simulink model "flightController"  (R2022a)
settings: Solver=ode3  StartTime=0  StopTime=TFinal  FixedStep=Ts  RelTol=1e-3  EnableMultiTasking=on
undefined symbols (not defined in the file): Controller, DiscIntNeverNeededParam, Ts, Vehicle
libraries: vrlib x2, dspfdesign x1
(part 1 of 2)
settings Model: Creator=The MathWorks, Inc.  LastModifiedBy=martin
settings SolverCC: AlgebraicLoopSolver=TrustRegion  MinimalZcImpactIntegration=on
settings DataIOCC: LimitDataPoints=on  SaveFormat=Array  ReturnWorkspaceOutputs=off
settings OptimizationCC: BlockReduction=off  DefaultParameterBehavior=Inlined  BufferReuse=off  PassReuseOutputArgsThreshold=0
settings DebuggingCC: AlgebraicLoopMsg=none  ParameterPrecisionLossMsg=none  ParameterTunabilityLossMsg=error  BusObjectLabelMismatch=error  SFUnexpectedBacktrackingDiag=warning  SFNoUnconditionalDefaultTransitionDiag=warning  SFExecutionAtInitializationDiag=none  SFMachineParentedDataDiag=warning  ArithmeticOperatorsInVariantConditions=warning
settings HardwareCC: ProdBitPerPointer=32  ProdBitPerSizeT=32  ProdBitPerPtrDiffT=32  ProdLargestAtomicInteger=Long  ProdWordSize=32  ProdHWDeviceType=ARM Compatible->ARM 9
settings ModelReferenceCC: ModelReferenceNumInstancesAllowed=Single  PropagateSignalLabelsOutOfModel=off
settings SFSimCC: SimUseLocalCustomCode=off  CustomCodeUndefinedFunction=UseInterfaceOnly
settings RTWCC: Description=Generic Real-Time Target  GenerateReport=on  RTWUseLocalCustomCode=off  LaunchReport=on  DLArmComputeVersion=19.05
settings CodeAppCC: ForceParamTrailComments=on  MaxIdLength=63  OperatorAnnotations=on  StateflowObjectComments=on  MATLABSourceComments=on
settings GRTTargetCC: TargetLangStandard=C89/C90 (ANSI)
settings ConfigComp: CovMetricSettings=dw  CovSaveCumulativeToWorkspaceVar=on  CovSaveSingleToWorkspaceVar=on  CovExternalEMLEnable=off  CovSFcnEnable=off

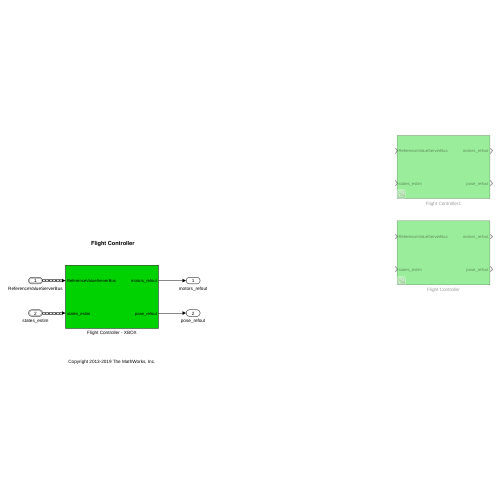
[thumbnail: Simulink's stored preview of the top-level diagram]
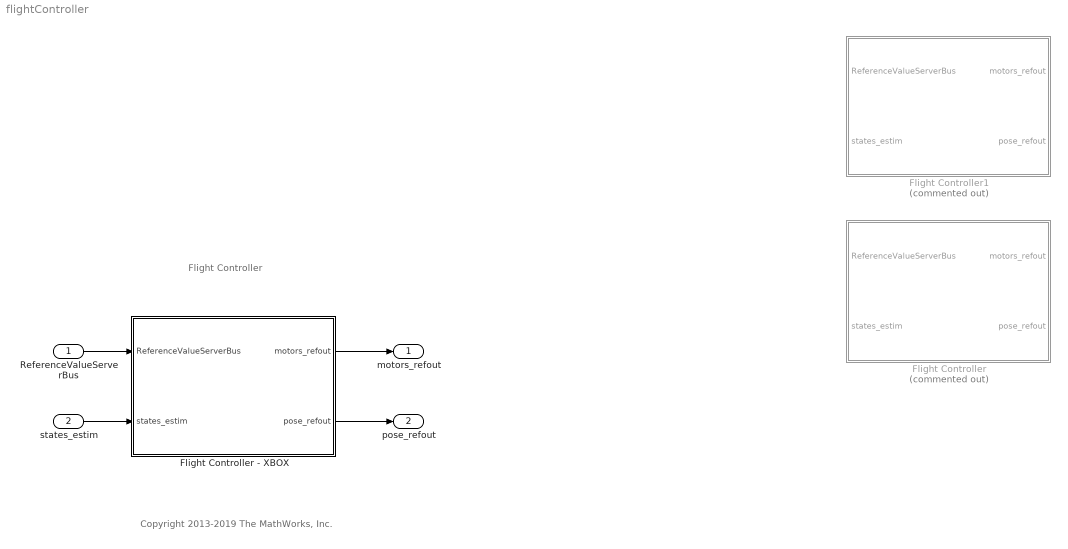
== system flightController ==
  note: Flight Controller
  note: Copyright 2013-2019 The MathWorks, Inc.
  ReferenceValueServerBus : Inport  OutDataTypeStr=Bus: CommandBus  BusOutputAsStruct=on
  states_estim : Inport  Port=2  OutDataTypeStr=Bus: statesEstim_t  BusOutputAsStruct=on
  Flight Controller : Subsystem  Commented=on
  Flight Controller - XBOX : Subsystem
  Flight Controller1 : Subsystem  Commented=on
  motors_refout : Outport  VectorParamsAs1DForOutWhenUnconnected=off
  pose_refout : Outport  Port=2  VectorParamsAs1DForOutWhenUnconnected=off
  wires:
  ReferenceValueServerBus/1 -> Flight Controller - XBOX/1(ReferenceValueServerBus)
  states_estim/1 -> Flight Controller - XBOX/2(states_estim)
  Flight Controller - XBOX/2(pose_refout) -> pose_refout/1
  Flight Controller - XBOX/1(motors_refout) -> motors_refout/1

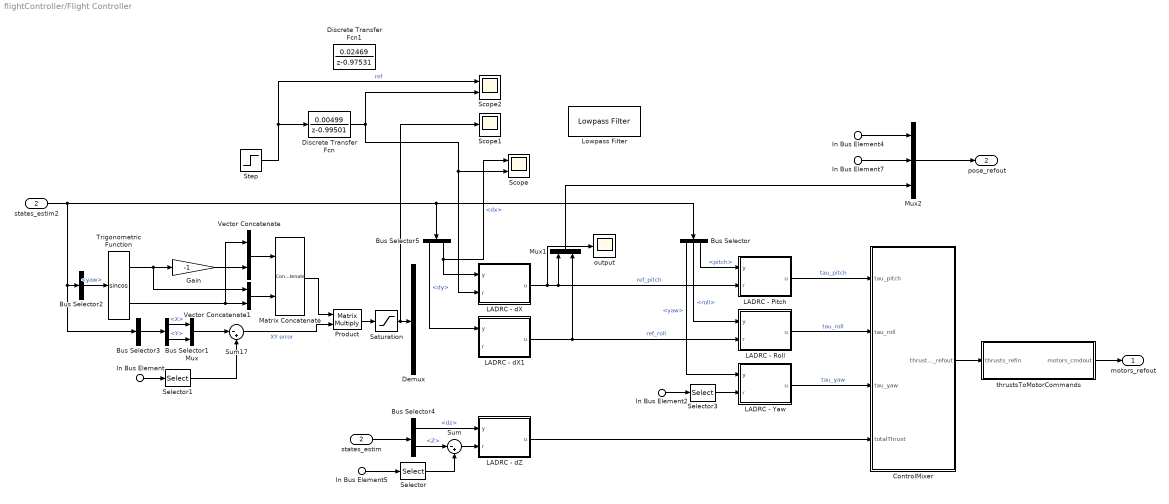
== system flightController/Flight Controller ==
  In Bus Element4 : Inport  PortName=ReferenceValueServerBus  Element=pos_ref
  In Bus Element5 : Inport  PortName=ReferenceValueServerBus  Element=pos_ref
  In Bus Element : Inport  PortName=ReferenceValueServerBus  Element=pos_ref
  In Bus Element2 : Inport  PortName=ReferenceValueServerBus  Element=orient_ref
  In Bus Element7 : Inport  PortName=ReferenceValueServerBus  Element=orient_ref
  states_estim : Inport  Port=2
  Bus Selector : BusSelector  OutputSignals=yaw,roll,pitch
  Bus Selector1 : BusSelector  OutputSignals=X,Y
  Bus Selector2 : BusSelector  OutputSignals=yaw
  Bus Selector3 : BusSelector  OutputSignals=X,Y  OutputAsBus=on
  Bus Selector4 : BusSelector  OutputSignals=dz,Z
  Bus Selector5 : BusSelector  OutputSignals=dy,dx
  ControlMixer : Subsystem
  Demux : Demux  Outputs=2
  Discrete Transfer Fcn : DiscreteTransferFcn  Numerator=[0.00499]  Denominator=[1 -0.99501]
  Discrete Transfer Fcn1 : DiscreteTransferFcn  Numerator=[0.02469]  Denominator=[1 -0.97531]
  Gain : Gain  Gain=-1
  LADRC - Pitch : Subsystem  VariantControl=Choice
  LADRC - Roll : Subsystem  VariantControl=Choice
  LADRC - Yaw : Subsystem  VariantControl=Choice
  LADRC - dX : Subsystem  VariantControl=Choice
  LADRC - dX1 : Subsystem  VariantControl=Choice
  LADRC - dZ : Subsystem  VariantControl=Choice
  Lowpass Filter : dspfdesign/Lowpass Filter  FilterType=IIR  DesignForMinimumOrder=off  FilterOrder=1  PassbandFrequency=4  StopbandFrequency=12e3  PassbandRipple=0.1  StopbandAttenuation=80  InheritSampleRate=off  SampleRate=200  SimulateUsing=Interpreted execution  roundingMode=Floor  coeffsDataTypeStr=fixdt(1,16)
  Matrix Concatenate : Concatenate  Mode=Multidimensional array  ConcatenateDimension=2
  Mux : Mux  Inputs=2
  Mux1 : Mux  Inputs=2
  Mux2 : Mux  Inputs=3
  Product : Product  Multiplication=Matrix(*)  OutDataTypeStr=single  RndMeth=Zero
  Saturation : Saturate  UpperLimit=3  LowerLimit=-3  OutDataTypeStr=single
  Scope : Scope  NumInputPorts=2
  Scope1 : Scope
  Scope2 : Scope  NumInputPorts=2
  Selector : Selector  InputPortWidth=3  IndexOptions=Index vector (dialog)  Indices=3  OutputSizes=1
  Selector1 : Selector  InputPortWidth=3  IndexOptions=Index vector (dialog)  Indices=[1 2]  OutputSizes=1
  Selector3 : Selector  InputPortWidth=3  IndexOptions=Index vector (dialog)  Indices=1  OutputSizes=1
  Step : Step  Time=5  After=0.5  SampleTime=Ts
  Sum : Sum  Inputs=|-+
  Sum17 : Sum  Inputs=|-+  AccumDataTypeStr=single
  Trigonometric Function : Trigonometry  Operator=sincos
  Vector Concatenate : Concatenate
  Vector Concatenate1 : Concatenate
  output : Scope
  states_estim2 : InportShadow  Port=2
  thrustsToMotorCommands : Subsystem
  motors_refout : Outport  VectorParamsAs1DForOutWhenUnconnected=off
  pose_refout : Outport  Port=2  VectorParamsAs1DForOutWhenUnconnected=off
  wires:
  thrustsToMotorCommands/1(motors_cmdout) -> motors_refout/1
  Mux2/1 -> pose_refout/1
  LADRC - dZ/1(u) -> ControlMixer/4(totalThrust)
  In Bus Element2/1 -> Selector3/1
  ControlMixer/1(thrusts_refout) -> thrustsToMotorCommands/1(thrusts_refin)
  Bus Selector5/2 -> Scope/1, LADRC - dX/1(y)  "<dx>"
  Bus Selector5/1 -> LADRC - dX1/1(y)  "<dy>"
  In Bus Element7/1 -> Mux2/2
  Selector3/1 -> LADRC - Yaw/2(r)
  Bus Selector4/1 -> LADRC - dZ/1(y)  "<dz>"
  In Bus Element5/1 -> Selector/1
  In Bus Element4/1 -> Mux2/1
  states_estim/1 -> Bus Selector4/1
  LADRC - Yaw/1(u) -> ControlMixer/3(tau_yaw)  "tau_yaw"
  Bus Selector/2 -> LADRC - Roll/1(y)  "<roll>"
  Bus Selector/3 -> LADRC - Pitch/1(y)  "<pitch>"
  LADRC - dX/1(u) -> output/1, LADRC - Pitch/2(r), Mux1/1  "ref_pitch"
  LADRC - Roll/1(u) -> ControlMixer/2(tau_roll)  "tau_roll"
  LADRC - dX1/1(u) -> LADRC - Roll/2(r), Mux1/2  "ref_roll"
  Mux1/1 -> Mux2/3
  LADRC - Pitch/1(u) -> ControlMixer/1(tau_pitch)  "tau_pitch"
  Bus Selector/1 -> LADRC - Yaw/1(y)  "<yaw>"
  Sum/1 -> LADRC - dZ/2(r)
  Bus Selector4/2 -> Sum/1  "<Z>"
  Selector/1 -> Sum/2
  Trigonometric Function/1 -> Gain/1, Vector Concatenate1/1
  Bus Selector3/1 -> Bus Selector1/1
  Bus Selector1/2 -> Mux/2  "<Y>"
  Mux/1 -> Sum17/1
  Sum17/1 -> Product/2  "XY error"
  Matrix Concatenate/1 -> Product/1
  Trigonometric Function/2 -> Vector Concatenate1/2, Vector Concatenate/1
  Bus Selector1/1 -> Mux/1  "<X>"
  Vector Concatenate1/1 -> Matrix Concatenate/2
  Bus Selector2/1 -> Trigonometric Function/1  "<yaw>"
  Gain/1 -> Vector Concatenate/2
  Product/1 -> Saturation/1
  Vector Concatenate/1 -> Matrix Concatenate/1
  states_estim2/1 -> Bus Selector/1, Bus Selector5/1, Bus Selector2/1, Bus Selector3/1
  In Bus Element/1 -> Selector1/1
  Selector1/1 -> Sum17/2
  Saturation/1 -> Scope1/1, Demux/1
  Step/1 -> Scope2/1, Discrete Transfer Fcn/1  "ref"
  ? -> LADRC - dX1/2(r)
  Discrete Transfer Fcn/1 -> Scope/2, LADRC - dX/2(r), Scope2/2

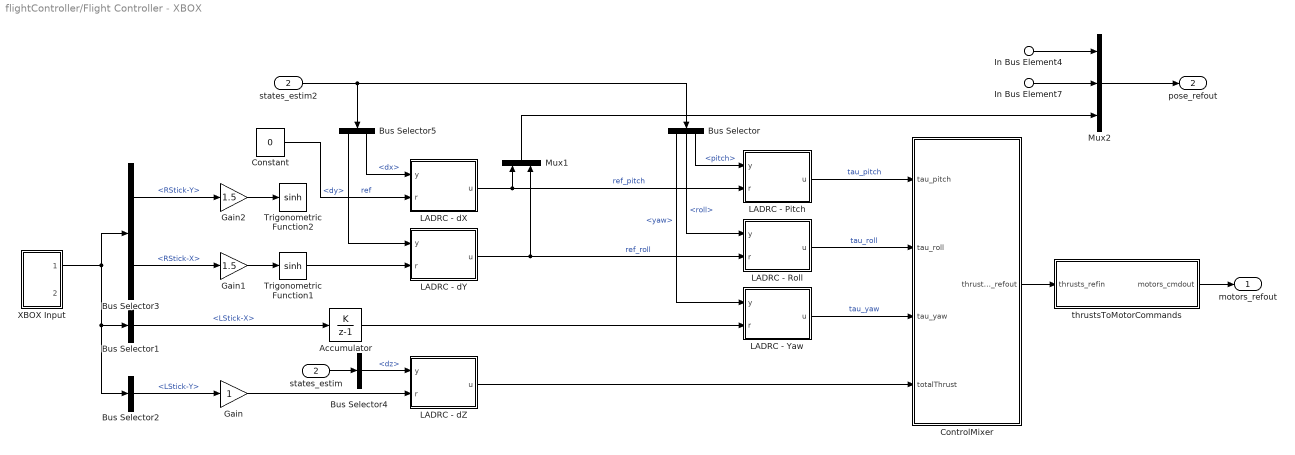
== system flightController/Flight Controller - XBOX ==
  In Bus Element4 : Inport  PortName=ReferenceValueServerBus  Element=pos_ref
  In Bus Element7 : Inport  PortName=ReferenceValueServerBus  Element=orient_ref
  states_estim : Inport  Port=2
  Accumulator : DiscreteIntegrator  IntegratorMethod=Accumulation: Forward Euler  gainval=0.01  SampleTime=-1  ICPrevOutput=DiscIntNeverNeededParam  ICPrevScaledInput=DiscIntNeverNeededParam
  Bus Selector : BusSelector  OutputSignals=yaw,roll,pitch
  Bus Selector1 : BusSelector  OutputSignals=LStick-X
  Bus Selector2 : BusSelector  OutputSignals=LStick-Y
  Bus Selector3 : BusSelector  OutputSignals=RStick-Y,RStick-X
  Bus Selector4 : BusSelector  OutputSignals=dz
  Bus Selector5 : BusSelector  OutputSignals=dy,dx
  Constant : Constant  Value=0  OutDataTypeStr=single  SampleTime=Ts
  ControlMixer : Subsystem
  Gain : Gain  OutDataTypeStr=single
  Gain1 : Gain  Gain=1.5  OutDataTypeStr=single
  Gain2 : Gain  Gain=1.5  OutDataTypeStr=single
  LADRC - Pitch : Subsystem  VariantControl=Choice
  LADRC - Roll : Subsystem  VariantControl=Choice
  LADRC - Yaw : Subsystem  VariantControl=Choice
  LADRC - dX : Subsystem  VariantControl=Choice
  LADRC - dY : Subsystem  VariantControl=Choice
  LADRC - dZ : Subsystem  VariantControl=Choice
  Mux1 : Mux  Inputs=2
  Mux2 : Mux  Inputs=3
  Trigonometric Function1 : Trigonometry  Operator=sinh
  Trigonometric Function2 : Trigonometry  Operator=sinh
  XBOX Input : Subsystem
  states_estim2 : InportShadow  Port=2
  thrustsToMotorCommands : Subsystem
  motors_refout : Outport  VectorParamsAs1DForOutWhenUnconnected=off
  pose_refout : Outport  Port=2  VectorParamsAs1DForOutWhenUnconnected=off
  wires:
  XBOX Input/1(Analog) -> Bus Selector3/1, Bus Selector2/1, Bus Selector1/1
  thrustsToMotorCommands/1(motors_cmdout) -> motors_refout/1
  Mux2/1 -> pose_refout/1
  ControlMixer/1(thrusts_refout) -> thrustsToMotorCommands/1(thrusts_refin)
  Constant/1 -> LADRC - dX/2(r)  "ref"
  Bus Selector3/2 -> Gain1/1  "<RStick-X>"
  Bus Selector5/2 -> LADRC - dX/1(y)  "<dx>"
  Gain2/1 -> Trigonometric Function2/1
  Bus Selector3/1 -> Gain2/1  "<RStick-Y>"
  Bus Selector5/1 -> LADRC - dY/1(y)  "<dy>"
  Accumulator/1 -> LADRC - Yaw/2(r)
  In Bus Element7/1 -> Mux2/2
  Bus Selector4/1 -> LADRC - dZ/1(y)  "<dz>"
  Bus Selector2/1 -> Gain/1  "<LStick-Y>"
  Gain1/1 -> Trigonometric Function1/1
  In Bus Element4/1 -> Mux2/1
  Bus Selector1/1 -> Accumulator/1  "<LStick-X>"
  LADRC - Yaw/1(u) -> ControlMixer/3(tau_yaw)  "tau_yaw"
  Bus Selector/2 -> LADRC - Roll/1(y)  "<roll>"
  Bus Selector/3 -> LADRC - Pitch/1(y)  "<pitch>"
  LADRC - dX/1(u) -> LADRC - Pitch/2(r), Mux1/1  "ref_pitch"
  LADRC - Roll/1(u) -> ControlMixer/2(tau_roll)  "tau_roll"
  LADRC - dY/1(u) -> LADRC - Roll/2(r), Mux1/2  "ref_roll"
  Mux1/1 -> Mux2/3
  states_estim2/1 -> Bus Selector/1, Bus Selector5/1
  LADRC - Pitch/1(u) -> ControlMixer/1(tau_pitch)  "tau_pitch"
  Bus Selector/1 -> LADRC - Yaw/1(y)  "<yaw>"
  states_estim/1 -> Bus Selector4/1
  LADRC - dZ/1(u) -> ControlMixer/4(totalThrust)
  Trigonometric Function1/1 -> LADRC - dY/2(r)
  Gain/1 -> LADRC - dZ/2(r)

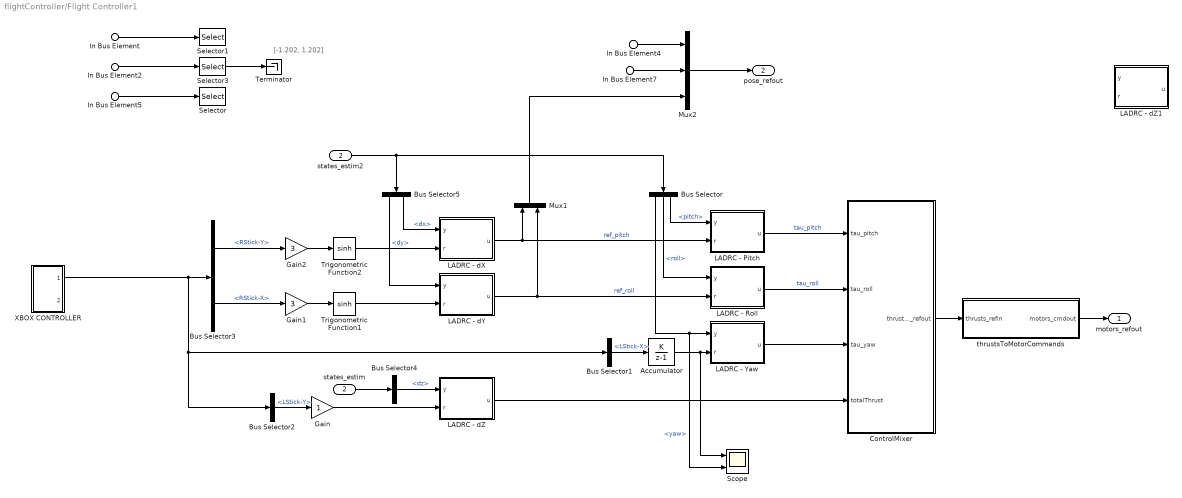
== system flightController/Flight Controller1 ==
  note: [-1.202, 1.202]
  In Bus Element : Inport  PortName=ReferenceValueServerBus  Element=pos_ref
  In Bus Element4 : Inport  PortName=ReferenceValueServerBus  Element=pos_ref
  In Bus Element5 : Inport  PortName=ReferenceValueServerBus  Element=pos_ref
  In Bus Element2 : Inport  PortName=ReferenceValueServerBus  Element=orient_ref
  In Bus Element7 : Inport  PortName=ReferenceValueServerBus  Element=orient_ref
  states_estim : Inport  Port=2
  Accumulator : DiscreteIntegrator  IntegratorMethod=Accumulation: Forward Euler  gainval=0.01  SampleTime=-1  ICPrevOutput=DiscIntNeverNeededParam  ICPrevScaledInput=DiscIntNeverNeededParam
  Bus Selector : BusSelector  OutputSignals=yaw,roll,pitch
  Bus Selector1 : BusSelector  OutputSignals=LStick-X
  Bus Selector2 : BusSelector  OutputSignals=LStick-Y
  Bus Selector3 : BusSelector  OutputSignals=RStick-Y,RStick-X
  Bus Selector4 : BusSelector  OutputSignals=dz
  Bus Selector5 : BusSelector  OutputSignals=dy,dx
  ControlMixer : Subsystem
  Gain : Gain  OutDataTypeStr=single
  Gain1 : Gain  Gain=3  OutDataTypeStr=single
  Gain2 : Gain  Gain=3  OutDataTypeStr=single
  LADRC - Pitch : Subsystem  VariantControl=Choice
  LADRC - Roll : Subsystem  VariantControl=Choice
  LADRC - Yaw : Subsystem  VariantControl=Choice
  LADRC - dX : Subsystem  VariantControl=Choice
  LADRC - dY : Subsystem  VariantControl=Choice
  LADRC - dZ : Subsystem  VariantControl=Choice
  LADRC - dZ1 : Subsystem  VariantControl=Choice
  Mux1 : Mux  Inputs=2
  Mux2 : Mux  Inputs=3
  Scope : Scope  NumInputPorts=2
  Selector : Selector  InputPortWidth=3  IndexOptions=Index vector (dialog)  Indices=3  OutputSizes=1
  Selector1 : Selector  InputPortWidth=3  IndexOptions=Index vector (dialog)  Indices=[1 2]  OutputSizes=1
  Selector3 : Selector  InputPortWidth=3  IndexOptions=Index vector (dialog)  Indices=1  OutputSizes=1
  Terminator : Terminator
  Trigonometric Function1 : Trigonometry  Operator=sinh
  Trigonometric Function2 : Trigonometry  Operator=sinh
  XBOX CONTROLLER : Subsystem
  states_estim2 : InportShadow  Port=2
  thrustsToMotorCommands : Subsystem
  motors_refout : Outport  VectorParamsAs1DForOutWhenUnconnected=off
  pose_refout : Outport  Port=2  VectorParamsAs1DForOutWhenUnconnected=off
  wires:
  XBOX CONTROLLER/1(Analog) -> Bus Selector2/1, Bus Selector1/1, Bus Selector3/1
  thrustsToMotorCommands/1(motors_cmdout) -> motors_refout/1
  Mux2/1 -> pose_refout/1
  In Bus Element/1 -> Selector1/1
  LADRC - dZ/1(u) -> ControlMixer/4(totalThrust)
  In Bus Element2/1 -> Selector3/1
  ControlMixer/1(thrusts_refout) -> thrustsToMotorCommands/1(thrusts_refin)
  Trigonometric Function2/1 -> LADRC - dX/2(r)
  Bus Selector3/2 -> Gain1/1  "<RStick-X>"
  Bus Selector5/2 -> LADRC - dX/1(y)  "<dx>"
  Gain2/1 -> Trigonometric Function2/1
  Bus Selector3/1 -> Gain2/1  "<RStick-Y>"
  Trigonometric Function1/1 -> LADRC - dY/2(r)
  Bus Selector5/1 -> LADRC - dY/1(y)  "<dy>"
  Accumulator/1 -> LADRC - Yaw/2(r), Scope/1
  In Bus Element7/1 -> Mux2/2
  Selector3/1 -> Terminator/1
  Bus Selector4/1 -> LADRC - dZ/1(y)  "<dz>"
  Bus Selector2/1 -> Gain/1  "<LStick-Y>"
  In Bus Element5/1 -> Selector/1
  Gain1/1 -> Trigonometric Function1/1
  In Bus Element4/1 -> Mux2/1
  states_estim/1 -> Bus Selector4/1
  Bus Selector1/1 -> Accumulator/1  "<LStick-X>"
  LADRC - Yaw/1(u) -> ControlMixer/3(tau_yaw)
  Bus Selector/2 -> LADRC - Roll/1(y)  "<roll>"
  Bus Selector/3 -> LADRC - Pitch/1(y)  "<pitch>"
  LADRC - dX/1(u) -> LADRC - Pitch/2(r), Mux1/1  "ref_pitch"
  LADRC - Roll/1(u) -> ControlMixer/2(tau_roll)  "tau_roll"
  LADRC - dY/1(u) -> Mux1/2, LADRC - Roll/2(r)  "ref_roll"
  Mux1/1 -> Mux2/3
  states_estim2/1 -> Bus Selector/1, Bus Selector5/1
  LADRC - Pitch/1(u) -> ControlMixer/1(tau_pitch)  "tau_pitch"
  Bus Selector/1 -> LADRC - Yaw/1(y), Scope/2  "<yaw>"
  Gain/1 -> LADRC - dZ/2(r)

== system flightController/Flight Controller/ControlMixer ==
  tau_pitch : Inport
  tau_roll : Inport  Port=2
  tau_yaw : Inport  Port=3
  totalThrust : Inport  Port=4
  Mux2 : Mux
  Product : Product  Multiplication=Matrix(*)  RndMeth=Zero
  TorqueTotalThrustToThrustPerMotor : Constant  Value=Controller.Q2Ts  OutDataTypeStr=single
  thrusts_refout : Outport  VectorParamsAs1DForOutWhenUnconnected=off
  wires:
  Product/1 -> thrusts_refout/1
  tau_roll/1 -> Mux2/4
  tau_pitch/1 -> Mux2/3
  tau_yaw/1 -> Mux2/2
  totalThrust/1 -> Mux2/1
  TorqueTotalThrustToThrustPerMotor/1 -> Product/1
  Mux2/1 -> Product/2

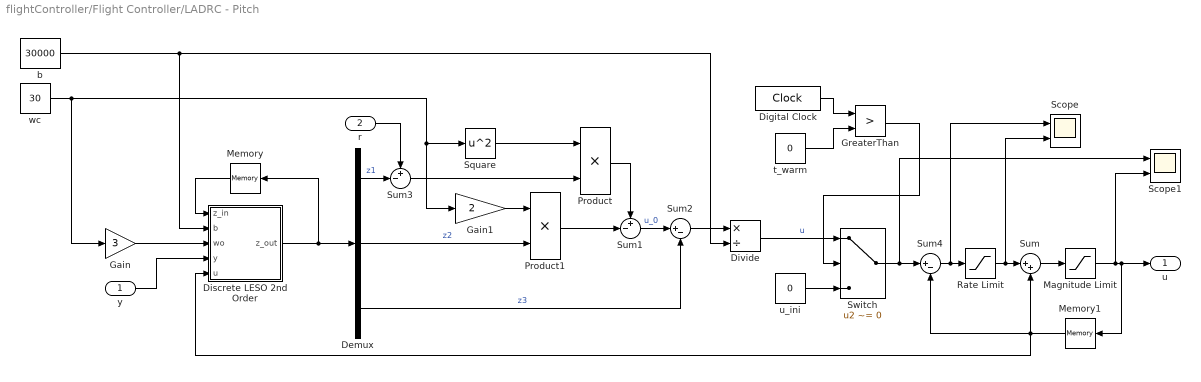
== system flightController/Flight Controller/LADRC - Pitch ==
  y : Inport
  r : Inport  Port=2
  Demux : Demux  Outputs=3
  Digital Clock : DigitalClock  SampleTime=Ts
  Discrete LESO 2nd Order : MATLAB Function  TreatAsAtomicUnit=on
  Divide : Product  Inputs=*/  OutDataTypeStr=single
  Gain : Gain  Gain=3  OutDataTypeStr=single
  Gain1 : Gain  Gain=2  OutDataTypeStr=single
  GreaterThan : RelationalOperator  Operator=>  OutDataTypeStr=boolean  RndMeth=Simplest  InputSameDT=off
  Magnitude Limit : Saturate  UpperLimit=4*Controller.totalThrustMaxRelative*Controller.motorsThrustPerMotorMax  LowerLimit=-4*Controller.totalThrustMaxRelative*Controller.motorsThrustPerMotorMax  OutDataTypeStr=single
  Memory : Memory  InitialCondition=[0 0 0]'
  Memory1 : Memory
  Product : Product  OutDataTypeStr=single
  Product1 : Product  OutDataTypeStr=single
  Rate Limit : Saturate  UpperLimit=0.05  LowerLimit=-0.05
  Scope : Scope  NumInputPorts=2
  Scope1 : Scope  NumInputPorts=2
  Square : Math  Operator=square
  Sum : Sum  Inputs=|++
  Sum1 : Sum  Inputs=+-|
  Sum2 : Sum  Inputs=|+-
  Sum3 : Sum  Inputs=+-|
  Sum4 : Sum  Inputs=|+-
  Switch : Switch  Criteria=u2 ~= 0  Threshold=0.1  SaturateOnIntegerOverflow=off  InputSameDT=off
  b : Constant  Value=30000  OutDataTypeStr=single
  t_warm : Constant  Value=0  OutDataTypeStr=single
  u_ini : Constant  Value=0  OutDataTypeStr=single
  wc : Constant  Value=30  OutDataTypeStr=single
  u : Outport
  wires:
  Discrete LESO 2nd Order/1(z_out) -> Memory/1, Demux/1
  Demux/1 -> Sum3/2  "z1"
  Product/1 -> Sum1/1
  Sum1/1 -> Sum2/1  "u_0"
  Demux/3 -> Sum2/2  "z3"
  Sum2/1 -> Divide/1
  Square/1 -> Product/1
  Gain1/1 -> Product1/1
  Demux/2 -> Product1/2  "z2"
  Product1/1 -> Sum1/2
  Divide/1 -> Switch/1  "u"
  u_ini/1 -> Switch/3
  r/1 -> Sum3/1
  Sum3/1 -> Product/2
  b/1 -> Divide/2, Discrete LESO 2nd Order/2(b)
  wc/1 -> Gain/1, Square/1, Gain1/1
  Gain/1 -> Discrete LESO 2nd Order/3(wo)
  t_warm/1 -> GreaterThan/2
  Digital Clock/1 -> GreaterThan/1
  GreaterThan/1 -> Switch/2
  y/1 -> Discrete LESO 2nd Order/4(y)
  Memory/1 -> Discrete LESO 2nd Order/1(z_in)
  Memory1/1 -> Sum4/2, Discrete LESO 2nd Order/5(u), Sum/2
  Rate Limit/1 -> Scope/2, Sum/1
  Sum/1 -> Magnitude Limit/1
  Sum4/1 -> Scope/1, Rate Limit/1
  Switch/1 -> Scope1/1, Sum4/1
  Magnitude Limit/1 -> Scope1/2, u/1, Memory1/1

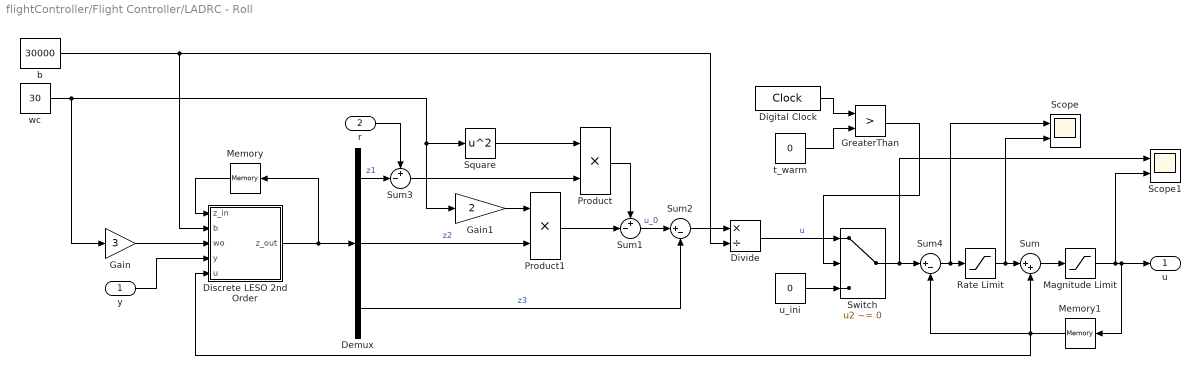
== system flightController/Flight Controller/LADRC - Roll ==
  y : Inport
  r : Inport  Port=2
  Demux : Demux  Outputs=3
  Digital Clock : DigitalClock  SampleTime=Ts
  Discrete LESO 2nd Order : MATLAB Function  TreatAsAtomicUnit=on
  Divide : Product  Inputs=*/  OutDataTypeStr=single
  Gain : Gain  Gain=3  OutDataTypeStr=single
  Gain1 : Gain  Gain=2  OutDataTypeStr=single
  GreaterThan : RelationalOperator  Operator=>  OutDataTypeStr=boolean  RndMeth=Simplest  InputSameDT=off
  Magnitude Limit : Saturate  UpperLimit=4*Controller.totalThrustMaxRelative*Controller.motorsThrustPerMotorMax  LowerLimit=-4*Controller.totalThrustMaxRelative*Controller.motorsThrustPerMotorMax  OutDataTypeStr=single
  Memory : Memory  InitialCondition=[0 0 0]'
  Memory1 : Memory
  Product : Product  OutDataTypeStr=single
  Product1 : Product  OutDataTypeStr=single
  Rate Limit : Saturate  UpperLimit=0.05  LowerLimit=-0.05
  Scope : Scope  NumInputPorts=2
  Scope1 : Scope  NumInputPorts=2
  Square : Math  Operator=square
  Sum : Sum  Inputs=|++
  Sum1 : Sum  Inputs=+-|
  Sum2 : Sum  Inputs=|+-
  Sum3 : Sum  Inputs=+-|
  Sum4 : Sum  Inputs=|+-
  Switch : Switch  Criteria=u2 ~= 0  Threshold=0.1  SaturateOnIntegerOverflow=off  InputSameDT=off
  b : Constant  Value=30000  OutDataTypeStr=single
  t_warm : Constant  Value=0  OutDataTypeStr=single
  u_ini : Constant  Value=0  OutDataTypeStr=single
  wc : Constant  Value=30  OutDataTypeStr=single
  u : Outport
  wires:
  Discrete LESO 2nd Order/1(z_out) -> Memory/1, Demux/1
  Demux/1 -> Sum3/2  "z1"
  Product/1 -> Sum1/1
  Sum1/1 -> Sum2/1  "u_0"
  Demux/3 -> Sum2/2  "z3"
  Sum2/1 -> Divide/1
  Square/1 -> Product/1
  Gain1/1 -> Product1/1
  Demux/2 -> Product1/2  "z2"
  Product1/1 -> Sum1/2
  Divide/1 -> Switch/1  "u"
  u_ini/1 -> Switch/3
  r/1 -> Sum3/1
  Sum3/1 -> Product/2
  b/1 -> Divide/2, Discrete LESO 2nd Order/2(b)
  wc/1 -> Gain/1, Square/1, Gain1/1
  Gain/1 -> Discrete LESO 2nd Order/3(wo)
  t_warm/1 -> GreaterThan/2
  Digital Clock/1 -> GreaterThan/1
  GreaterThan/1 -> Switch/2
  y/1 -> Discrete LESO 2nd Order/4(y)
  Memory/1 -> Discrete LESO 2nd Order/1(z_in)
  Memory1/1 -> Sum4/2, Discrete LESO 2nd Order/5(u), Sum/2
  Rate Limit/1 -> Scope/2, Sum/1
  Sum/1 -> Magnitude Limit/1
  Sum4/1 -> Scope/1, Rate Limit/1
  Switch/1 -> Scope1/1, Sum4/1
  Magnitude Limit/1 -> Scope1/2, u/1, Memory1/1

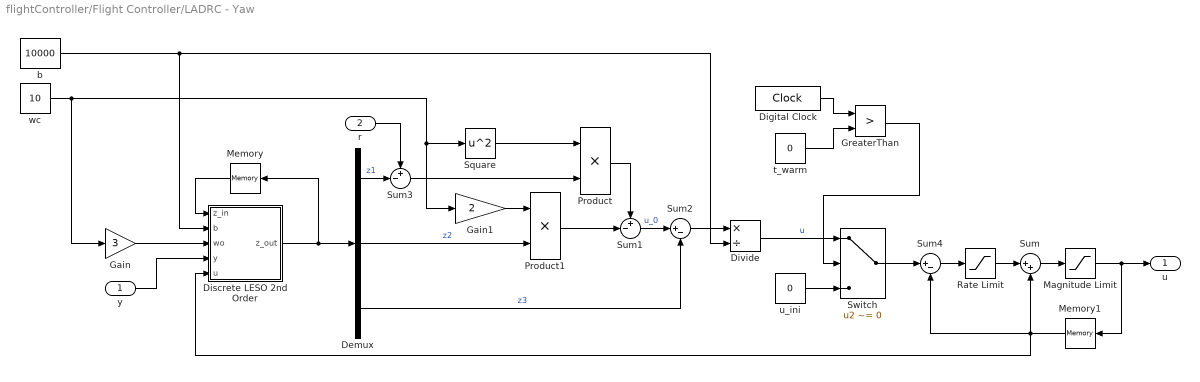
== system flightController/Flight Controller/LADRC - Yaw ==
  y : Inport
  r : Inport  Port=2
  Demux : Demux  Outputs=3
  Digital Clock : DigitalClock  SampleTime=Ts
  Discrete LESO 2nd Order : MATLAB Function  TreatAsAtomicUnit=on
  Divide : Product  Inputs=*/  OutDataTypeStr=single
  Gain : Gain  Gain=3  OutDataTypeStr=single
  Gain1 : Gain  Gain=2  OutDataTypeStr=single
  GreaterThan : RelationalOperator  Operator=>  OutDataTypeStr=boolean  RndMeth=Simplest  InputSameDT=off
  Magnitude Limit : Saturate  UpperLimit=4*Controller.totalThrustMaxRelative*Controller.motorsThrustPerMotorMax  LowerLimit=-4*Controller.totalThrustMaxRelative*Controller.motorsThrustPerMotorMax  OutDataTypeStr=single
  Memory : Memory  InitialCondition=[0 0 0]'
  Memory1 : Memory
  Product : Product  OutDataTypeStr=single
  Product1 : Product  OutDataTypeStr=single
  Rate Limit : Saturate  UpperLimit=0.05  LowerLimit=-0.05
  Square : Math  Operator=square
  Sum : Sum  Inputs=|++
  Sum1 : Sum  Inputs=+-|
  Sum2 : Sum  Inputs=|+-
  Sum3 : Sum  Inputs=+-|
  Sum4 : Sum  Inputs=|+-
  Switch : Switch  Criteria=u2 ~= 0  Threshold=0.1  SaturateOnIntegerOverflow=off  InputSameDT=off
  b : Constant  Value=10000  OutDataTypeStr=single
  t_warm : Constant  Value=0  OutDataTypeStr=single
  u_ini : Constant  Value=0  OutDataTypeStr=single
  wc : Constant  Value=10  OutDataTypeStr=single
  u : Outport
  wires:
  Discrete LESO 2nd Order/1(z_out) -> Memory/1, Demux/1
  Demux/1 -> Sum3/2  "z1"
  Product/1 -> Sum1/1
  Sum1/1 -> Sum2/1  "u_0"
  Demux/3 -> Sum2/2  "z3"
  Sum2/1 -> Divide/1
  Square/1 -> Product/1
  Gain1/1 -> Product1/1
  Demux/2 -> Product1/2  "z2"
  Product1/1 -> Sum1/2
  Divide/1 -> Switch/1  "u"
  u_ini/1 -> Switch/3
  r/1 -> Sum3/1
  Sum3/1 -> Product/2
  b/1 -> Divide/2, Discrete LESO 2nd Order/2(b)
  wc/1 -> Gain/1, Square/1, Gain1/1
  Gain/1 -> Discrete LESO 2nd Order/3(wo)
  t_warm/1 -> GreaterThan/2
  Digital Clock/1 -> GreaterThan/1
  GreaterThan/1 -> Switch/2
  y/1 -> Discrete LESO 2nd Order/4(y)
  Memory/1 -> Discrete LESO 2nd Order/1(z_in)
  Memory1/1 -> Sum4/2, Discrete LESO 2nd Order/5(u), Sum/2
  Rate Limit/1 -> Sum/1
  Sum/1 -> Magnitude Limit/1
  Sum4/1 -> Rate Limit/1
  Switch/1 -> Sum4/1
  Magnitude Limit/1 -> u/1, Memory1/1

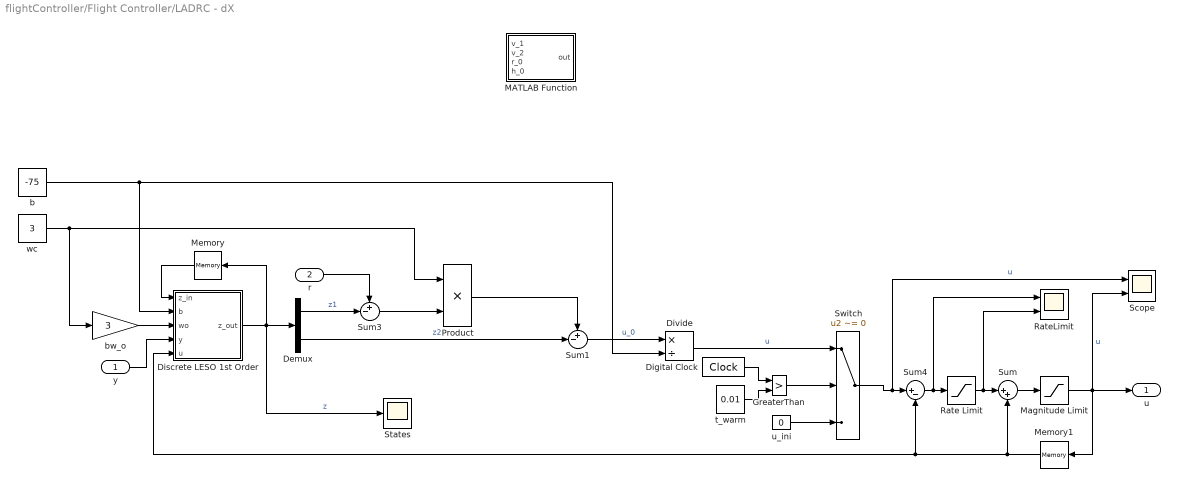
== system flightController/Flight Controller/LADRC - dX ==
  y : Inport
  r : Inport  Port=2
  Demux : Demux  Outputs=2
  Digital Clock : DigitalClock  SampleTime=Ts
  Discrete LESO 1st Order : MATLAB Function  TreatAsAtomicUnit=on
  Divide : Product  Inputs=*/
  GreaterThan : RelationalOperator  Operator=>  OutDataTypeStr=boolean  RndMeth=Simplest  InputSameDT=off
  MATLAB Function : MATLAB Function  TreatAsAtomicUnit=on
  Magnitude Limit : Saturate  UpperLimit=pi/8  LowerLimit=-pi/8  OutDataTypeStr=single
  Memory : Memory  InitialCondition=[0 0]'
  Memory1 : Memory
  Product : Product
  Rate Limit : Saturate  UpperLimit=0.2  LowerLimit=-0.2
  RateLimit : Scope  NumInputPorts=2
  Scope : Scope  NumInputPorts=2
  States : Scope
  Sum : Sum  Inputs=|++
  Sum1 : Sum  Inputs=+-|
  Sum3 : Sum  Inputs=+-|
  Sum4 : Sum  Inputs=|+-
  Switch : Switch  Criteria=u2 ~= 0  Threshold=0.1  SaturateOnIntegerOverflow=off  InputSameDT=off
  b : Constant  Value=-75  OutDataTypeStr=single
  bw_o : Gain  Gain=3
  t_warm : Constant  Value=0.01
  u_ini : Constant  Value=0  OutDataTypeStr=single
  wc : Constant  Value=3  OutDataTypeStr=single
  u : Outport
  wires:
  Demux/1 -> Sum3/2  "z1"
  Product/1 -> Sum1/1
  Sum1/1 -> Divide/1  "u_0"
  Demux/2 -> Sum1/2  "z2"
  Magnitude Limit/1 -> Scope/2, u/1, Memory1/1  "u"
  Divide/1 -> Switch/1  "u"
  u_ini/1 -> Switch/3
  r/1 -> Sum3/1
  Sum3/1 -> Product/2
  b/1 -> Divide/2, Discrete LESO 1st Order/2(b)
  wc/1 -> Product/1, bw_o/1
  bw_o/1 -> Discrete LESO 1st Order/3(wo)
  t_warm/1 -> GreaterThan/2
  Digital Clock/1 -> GreaterThan/1
  GreaterThan/1 -> Switch/2
  y/1 -> Discrete LESO 1st Order/4(y)
  Switch/1 -> Scope/1, Sum4/1  "u"
  Discrete LESO 1st Order/1(z_out) -> States/1, Memory/1, Demux/1  "z"
  Memory/1 -> Discrete LESO 1st Order/1(z_in)
  Rate Limit/1 -> RateLimit/2, Sum/1
  Memory1/1 -> Discrete LESO 1st Order/5(u), Sum4/2, Sum/2
  Sum4/1 -> RateLimit/1, Rate Limit/1
  Sum/1 -> Magnitude Limit/1

== system flightController/Flight Controller/LADRC - dX1 ==
  y : Inport
  r : Inport  Port=2
  Demux : Demux  Outputs=2
  Digital Clock : DigitalClock  SampleTime=Ts
  Discrete LESO 1st Order : MATLAB Function  TreatAsAtomicUnit=on
  Divide : Product  Inputs=*/
  GreaterThan : RelationalOperator  Operator=>  OutDataTypeStr=boolean  RndMeth=Simplest  InputSameDT=off
  Magnitude Limit : Saturate  UpperLimit=pi/8  LowerLimit=-pi/8  OutDataTypeStr=single
  Memory : Memory  InitialCondition=[0 0]'
  Memory1 : Memory
  Product : Product
  Rate Limit : Saturate  UpperLimit=1  LowerLimit=-1
  Sum : Sum  Inputs=|++
  Sum1 : Sum  Inputs=+-|
  Sum3 : Sum  Inputs=+-|
  Sum4 : Sum  Inputs=|+-
  Switch : Switch  Criteria=u2 ~= 0  Threshold=0.1  SaturateOnIntegerOverflow=off  InputSameDT=off
  b : Constant  Value=60  OutDataTypeStr=single
  bw_o : Gain  Gain=3
  t_warm : Constant  Value=0.01
  u_ini : Constant  Value=0  OutDataTypeStr=single
  wc : Constant  OutDataTypeStr=single
  u : Outport
  wires:
  Demux/1 -> Sum3/2  "z1"
  Product/1 -> Sum1/1
  Sum1/1 -> Divide/1  "u_0"
  Demux/2 -> Sum1/2  "z2"
  Magnitude Limit/1 -> u/1, Memory1/1  "u"
  Divide/1 -> Switch/1  "u"
  u_ini/1 -> Switch/3
  r/1 -> Sum3/1
  Sum3/1 -> Product/2
  b/1 -> Divide/2, Discrete LESO 1st Order/2(b)
  wc/1 -> Product/1, bw_o/1
  bw_o/1 -> Discrete LESO 1st Order/3(wo)
  t_warm/1 -> GreaterThan/2
  Digital Clock/1 -> GreaterThan/1
  GreaterThan/1 -> Switch/2
  y/1 -> Discrete LESO 1st Order/4(y)
  Switch/1 -> Sum4/1  "u"
  Discrete LESO 1st Order/1(z_out) -> Memory/1, Demux/1
  Memory/1 -> Discrete LESO 1st Order/1(z_in)
  Rate Limit/1 -> Sum/1
  Memory1/1 -> Discrete LESO 1st Order/5(u), Sum4/2, Sum/2
  Sum4/1 -> Rate Limit/1
  Sum/1 -> Magnitude Limit/1

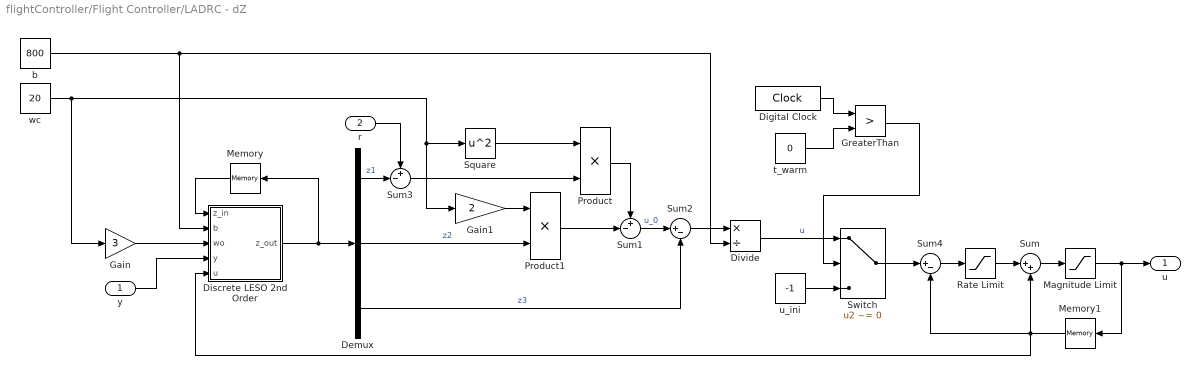
== system flightController/Flight Controller/LADRC - dZ ==
  y : Inport
  r : Inport  Port=2
  Demux : Demux  Outputs=3
  Digital Clock : DigitalClock  SampleTime=Ts
  Discrete LESO 2nd Order : MATLAB Function  TreatAsAtomicUnit=on
  Divide : Product  Inputs=*/  OutDataTypeStr=single
  Gain : Gain  Gain=3  OutDataTypeStr=single
  Gain1 : Gain  Gain=2  OutDataTypeStr=single
  GreaterThan : RelationalOperator  Operator=>  OutDataTypeStr=boolean  RndMeth=Simplest  InputSameDT=off
  Magnitude Limit : Saturate  UpperLimit=4*Controller.totalThrustMaxRelative*Controller.motorsThrustPerMotorMax  LowerLimit=-4*Controller.totalThrustMaxRelative*Controller.motorsThrustPerMotorMax  OutDataTypeStr=single
  Memory : Memory  InitialCondition=[0 0 380]'
  Memory1 : Memory  InitialCondition=-0.6
  Product : Product  OutDataTypeStr=single
  Product1 : Product  OutDataTypeStr=single
  Rate Limit : Saturate  UpperLimit=0.025  LowerLimit=-0.025
  Square : Math  Operator=square
  Sum : Sum  Inputs=|++
  Sum1 : Sum  Inputs=+-|
  Sum2 : Sum  Inputs=|+-
  Sum3 : Sum  Inputs=+-|
  Sum4 : Sum  Inputs=|+-
  Switch : Switch  Criteria=u2 ~= 0  Threshold=0.1  SaturateOnIntegerOverflow=off  InputSameDT=off
  b : Constant  Value=800  OutDataTypeStr=single
  t_warm : Constant  Value=0  OutDataTypeStr=single
  u_ini : Constant  Value=-1  OutDataTypeStr=single
  wc : Constant  Value=20  OutDataTypeStr=single
  u : Outport
  wires:
  Discrete LESO 2nd Order/1(z_out) -> Memory/1, Demux/1
  Demux/1 -> Sum3/2  "z1"
  Product/1 -> Sum1/1
  Sum1/1 -> Sum2/1  "u_0"
  Demux/3 -> Sum2/2  "z3"
  Sum2/1 -> Divide/1
  Square/1 -> Product/1
  Gain1/1 -> Product1/1
  Demux/2 -> Product1/2  "z2"
  Product1/1 -> Sum1/2
  Divide/1 -> Switch/1  "u"
  u_ini/1 -> Switch/3
  r/1 -> Sum3/1
  Sum3/1 -> Product/2
  b/1 -> Divide/2, Discrete LESO 2nd Order/2(b)
  wc/1 -> Gain/1, Square/1, Gain1/1
  Gain/1 -> Discrete LESO 2nd Order/3(wo)
  t_warm/1 -> GreaterThan/2
  Digital Clock/1 -> GreaterThan/1
  GreaterThan/1 -> Switch/2
  y/1 -> Discrete LESO 2nd Order/4(y)
  Memory/1 -> Discrete LESO 2nd Order/1(z_in)
  Memory1/1 -> Sum4/2, Discrete LESO 2nd Order/5(u), Sum/2
  Rate Limit/1 -> Sum/1
  Sum/1 -> Magnitude Limit/1
  Sum4/1 -> Rate Limit/1
  Switch/1 -> Sum4/1
  Magnitude Limit/1 -> u/1, Memory1/1

== system flightController/Flight Controller/thrustsToMotorCommands ==
  thrusts_refin : Inport
  1 : Constant  OutDataTypeStr=single
  10 : Constant  Value=10  OutDataTypeStr=single
  2 : Constant  Value=-1  OutDataTypeStr=single
  Digital Clock : DigitalClock  SampleTime=Ts
  Digital Clock1 : DigitalClock  SampleTime=Ts
  Gain : Gain  Gain=1/40  OutDataTypeStr=single
  GreaterThan : RelationalOperator  Operator=>  OutDataTypeStr=boolean  RndMeth=Simplest  InputSameDT=off
  MotorDirections : Gain  Gain=[1 -1 1 -1]
  Mux : Mux
  Product : Product  OutDataTypeStr=single
  Saturation : Saturate  UpperLimit=40  LowerLimit=0  OutDataTypeStr=single
  Saturation5 : Saturate  UpperLimit=Vehicle.Motor.maxLimit  LowerLimit=Vehicle.Motor.minLimit
  Scope : Scope
  Sum : Sum  Inputs=|+-
  Sum1 : Sum  Inputs=|-+
  Switch : Switch  Criteria=u2 ~= 0  Threshold=0.1  SaturateOnIntegerOverflow=off  InputSameDT=off
  ThrustToMotorCommand : Gain  Gain=-Vehicle.Motor.thrustToMotorCommand
  t_warm : Constant  Value=10  OutDataTypeStr=single
  motors_cmdout : Outport  VectorParamsAs1DForOutWhenUnconnected=off
  wires:
  Saturation5/1 -> Product/2, MotorDirections/1
  MotorDirections/1 -> Switch/3
  ThrustToMotorCommand/1 -> Saturation5/1
  thrusts_refin/1 -> ThrustToMotorCommand/1
  Product/1 -> Switch/1
  Switch/1 -> motors_cmdout/1
  GreaterThan/1 -> Switch/2
  Digital Clock/1 -> GreaterThan/1
  t_warm/1 -> GreaterThan/2
  Digital Clock1/1 -> Sum/1
  10/1 -> Sum/2
  Sum/1 -> Saturation/1
  Saturation/1 -> Gain/1
  1/1 -> Mux/3, Sum1/2
  2/1 -> Mux/2, Mux/4
  Sum1/1 -> Scope/1, Mux/1
  Mux/1 -> Product/1

== system flightController/Flight Controller - XBOX/ControlMixer ==
  tau_pitch : Inport
  tau_roll : Inport  Port=2
  tau_yaw : Inport  Port=3
  totalThrust : Inport  Port=4
  Mux2 : Mux
  Product : Product  Multiplication=Matrix(*)  RndMeth=Zero
  TorqueTotalThrustToThrustPerMotor : Constant  Value=Controller.Q2Ts  OutDataTypeStr=single
  thrusts_refout : Outport  VectorParamsAs1DForOutWhenUnconnected=off
  wires:
  Product/1 -> thrusts_refout/1
  tau_roll/1 -> Mux2/4
  tau_pitch/1 -> Mux2/3
  tau_yaw/1 -> Mux2/2
  totalThrust/1 -> Mux2/1
  TorqueTotalThrustToThrustPerMotor/1 -> Product/1
  Mux2/1 -> Product/2

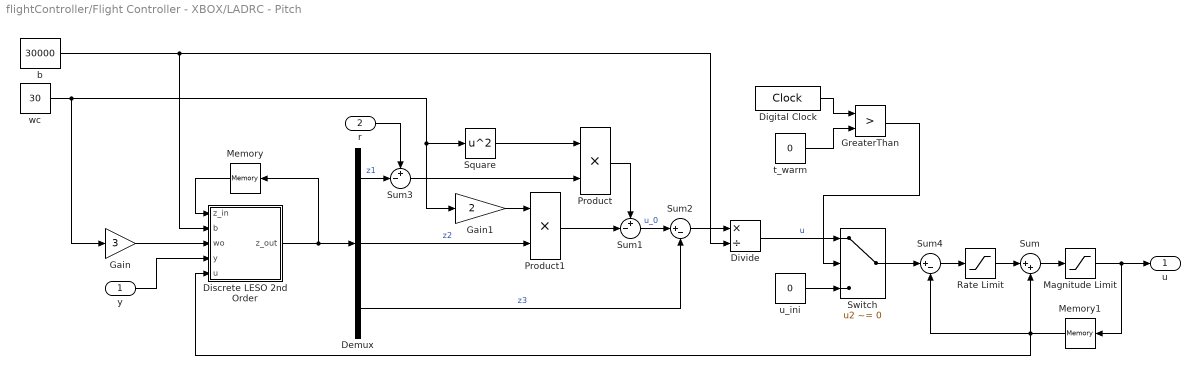
== system flightController/Flight Controller - XBOX/LADRC - Pitch ==
  y : Inport
  r : Inport  Port=2
  Demux : Demux  Outputs=3
  Digital Clock : DigitalClock  SampleTime=Ts
  Discrete LESO 2nd Order : MATLAB Function  TreatAsAtomicUnit=on
  Divide : Product  Inputs=*/  OutDataTypeStr=single
  Gain : Gain  Gain=3  OutDataTypeStr=single
  Gain1 : Gain  Gain=2  OutDataTypeStr=single
  GreaterThan : RelationalOperator  Operator=>  OutDataTypeStr=boolean  RndMeth=Simplest  InputSameDT=off
  Magnitude Limit : Saturate  UpperLimit=4*Controller.totalThrustMaxRelative*Controller.motorsThrustPerMotorMax  LowerLimit=-4*Controller.totalThrustMaxRelative*Controller.motorsThrustPerMotorMax  OutDataTypeStr=single
  Memory : Memory  InitialCondition=[0 0 0]'
  Memory1 : Memory
  Product : Product  OutDataTypeStr=single
  Product1 : Product  OutDataTypeStr=single
  Rate Limit : Saturate  UpperLimit=0.0001  LowerLimit=-0.0001
  Square : Math  Operator=square
  Sum : Sum  Inputs=|++
  Sum1 : Sum  Inputs=+-|
  Sum2 : Sum  Inputs=|+-
  Sum3 : Sum  Inputs=+-|
  Sum4 : Sum  Inputs=|+-
  Switch : Switch  Criteria=u2 ~= 0  Threshold=0.1  SaturateOnIntegerOverflow=off  InputSameDT=off
  b : Constant  Value=30000  OutDataTypeStr=single
  t_warm : Constant  Value=0  OutDataTypeStr=single
  u_ini : Constant  Value=0  OutDataTypeStr=single
  wc : Constant  Value=30  OutDataTypeStr=single
  u : Outport
  wires:
  Discrete LESO 2nd Order/1(z_out) -> Memory/1, Demux/1
  Demux/1 -> Sum3/2  "z1"
  Product/1 -> Sum1/1
  Sum1/1 -> Sum2/1  "u_0"
  Demux/3 -> Sum2/2  "z3"
  Sum2/1 -> Divide/1
  Square/1 -> Product/1
  Gain1/1 -> Product1/1
  Demux/2 -> Product1/2  "z2"
  Product1/1 -> Sum1/2
  Divide/1 -> Switch/1  "u"
  u_ini/1 -> Switch/3
  r/1 -> Sum3/1
  Sum3/1 -> Product/2
  b/1 -> Divide/2, Discrete LESO 2nd Order/2(b)
  wc/1 -> Gain/1, Square/1, Gain1/1
  Gain/1 -> Discrete LESO 2nd Order/3(wo)
  t_warm/1 -> GreaterThan/2
  Digital Clock/1 -> GreaterThan/1
  GreaterThan/1 -> Switch/2
  y/1 -> Discrete LESO 2nd Order/4(y)
  Memory/1 -> Discrete LESO 2nd Order/1(z_in)
  Memory1/1 -> Sum4/2, Discrete LESO 2nd Order/5(u), Sum/2
  Rate Limit/1 -> Sum/1
  Sum/1 -> Magnitude Limit/1
  Sum4/1 -> Rate Limit/1
  Switch/1 -> Sum4/1
  Magnitude Limit/1 -> u/1, Memory1/1

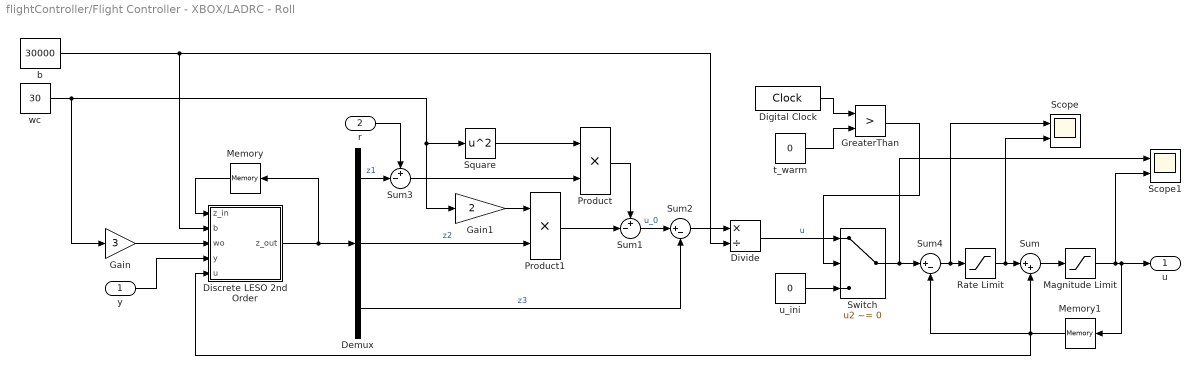
== system flightController/Flight Controller - XBOX/LADRC - Roll ==
  y : Inport
  r : Inport  Port=2
  Demux : Demux  Outputs=3
  Digital Clock : DigitalClock  SampleTime=Ts
  Discrete LESO 2nd Order : MATLAB Function  TreatAsAtomicUnit=on
  Divide : Product  Inputs=*/  OutDataTypeStr=single
  Gain : Gain  Gain=3  OutDataTypeStr=single
  Gain1 : Gain  Gain=2  OutDataTypeStr=single
  GreaterThan : RelationalOperator  Operator=>  OutDataTypeStr=boolean  RndMeth=Simplest  InputSameDT=off
  Magnitude Limit : Saturate  UpperLimit=4*Controller.totalThrustMaxRelative*Controller.motorsThrustPerMotorMax  LowerLimit=-4*Controller.totalThrustMaxRelative*Controller.motorsThrustPerMotorMax  OutDataTypeStr=single
  Memory : Memory  InitialCondition=[0 0 0]'
  Memory1 : Memory
  Product : Product  OutDataTypeStr=single
  Product1 : Product  OutDataTypeStr=single
  Rate Limit : Saturate  UpperLimit=0.0001  LowerLimit=-0.0001
  Scope : Scope  NumInputPorts=2
  Scope1 : Scope  NumInputPorts=2
  Square : Math  Operator=square
  Sum : Sum  Inputs=|++
  Sum1 : Sum  Inputs=+-|
  Sum2 : Sum  Inputs=|+-
  Sum3 : Sum  Inputs=+-|
  Sum4 : Sum  Inputs=|+-
  Switch : Switch  Criteria=u2 ~= 0  Threshold=0.1  SaturateOnIntegerOverflow=off  InputSameDT=off
  b : Constant  Value=30000  OutDataTypeStr=single
  t_warm : Constant  Value=0  OutDataTypeStr=single
  u_ini : Constant  Value=0  OutDataTypeStr=single
  wc : Constant  Value=30  OutDataTypeStr=single
  u : Outport
  wires:
  Discrete LESO 2nd Order/1(z_out) -> Memory/1, Demux/1
  Demux/1 -> Sum3/2  "z1"
  Product/1 -> Sum1/1
  Sum1/1 -> Sum2/1  "u_0"
  Demux/3 -> Sum2/2  "z3"
  Sum2/1 -> Divide/1
  Square/1 -> Product/1
  Gain1/1 -> Product1/1
  Demux/2 -> Product1/2  "z2"
  Product1/1 -> Sum1/2
  Divide/1 -> Switch/1  "u"
  u_ini/1 -> Switch/3
  r/1 -> Sum3/1
  Sum3/1 -> Product/2
  b/1 -> Divide/2, Discrete LESO 2nd Order/2(b)
  wc/1 -> Gain/1, Square/1, Gain1/1
  Gain/1 -> Discrete LESO 2nd Order/3(wo)
  t_warm/1 -> GreaterThan/2
  Digital Clock/1 -> GreaterThan/1
  GreaterThan/1 -> Switch/2
  y/1 -> Discrete LESO 2nd Order/4(y)
  Memory/1 -> Discrete LESO 2nd Order/1(z_in)
  Memory1/1 -> Sum4/2, Discrete LESO 2nd Order/5(u), Sum/2
  Rate Limit/1 -> Scope/2, Sum/1
  Sum/1 -> Magnitude Limit/1
  Sum4/1 -> Scope/1, Rate Limit/1
  Switch/1 -> Scope1/1, Sum4/1
  Magnitude Limit/1 -> Scope1/2, u/1, Memory1/1

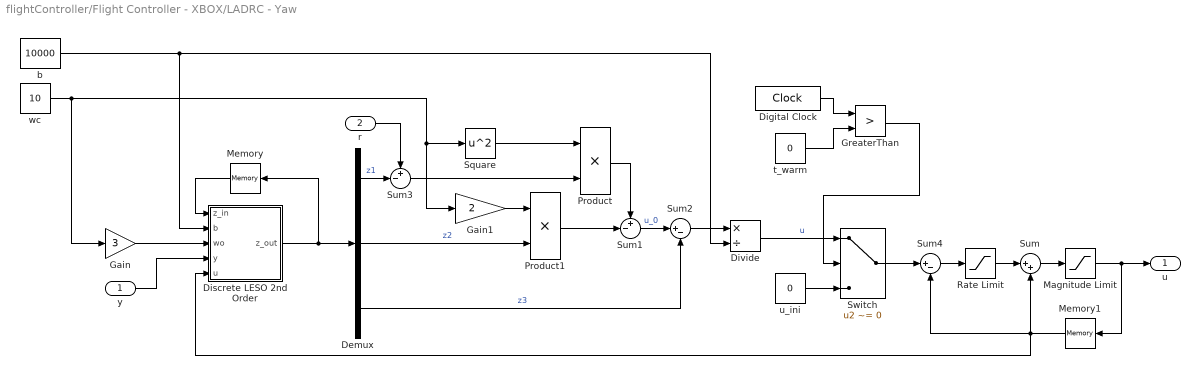
== system flightController/Flight Controller - XBOX/LADRC - Yaw ==
  y : Inport
  r : Inport  Port=2
  Demux : Demux  Outputs=3
  Digital Clock : DigitalClock  SampleTime=Ts
  Discrete LESO 2nd Order : MATLAB Function  TreatAsAtomicUnit=on
  Divide : Product  Inputs=*/  OutDataTypeStr=single
  Gain : Gain  Gain=3  OutDataTypeStr=single
  Gain1 : Gain  Gain=2  OutDataTypeStr=single
  GreaterThan : RelationalOperator  Operator=>  OutDataTypeStr=boolean  RndMeth=Simplest  InputSameDT=off
  Magnitude Limit : Saturate  UpperLimit=4*Controller.totalThrustMaxRelative*Controller.motorsThrustPerMotorMax  LowerLimit=-4*Controller.totalThrustMaxRelative*Controller.motorsThrustPerMotorMax  OutDataTypeStr=single
  Memory : Memory  InitialCondition=[0 0 0]'
  Memory1 : Memory
  Product : Product  OutDataTypeStr=single
  Product1 : Product  OutDataTypeStr=single
  Rate Limit : Saturate  UpperLimit=0.05  LowerLimit=-0.05
  Square : Math  Operator=square
  Sum : Sum  Inputs=|++
  Sum1 : Sum  Inputs=+-|
  Sum2 : Sum  Inputs=|+-
  Sum3 : Sum  Inputs=+-|
  Sum4 : Sum  Inputs=|+-
  Switch : Switch  Criteria=u2 ~= 0  Threshold=0.1  SaturateOnIntegerOverflow=off  InputSameDT=off
  b : Constant  Value=10000  OutDataTypeStr=single
  t_warm : Constant  Value=0  OutDataTypeStr=single
  u_ini : Constant  Value=0  OutDataTypeStr=single
  wc : Constant  Value=10  OutDataTypeStr=single
  u : Outport
  wires:
  Discrete LESO 2nd Order/1(z_out) -> Memory/1, Demux/1
  Demux/1 -> Sum3/2  "z1"
  Product/1 -> Sum1/1
  Sum1/1 -> Sum2/1  "u_0"
  Demux/3 -> Sum2/2  "z3"
  Sum2/1 -> Divide/1
  Square/1 -> Product/1
  Gain1/1 -> Product1/1
  Demux/2 -> Product1/2  "z2"
  Product1/1 -> Sum1/2
  Divide/1 -> Switch/1  "u"
  u_ini/1 -> Switch/3
  r/1 -> Sum3/1
  Sum3/1 -> Product/2
  b/1 -> Divide/2, Discrete LESO 2nd Order/2(b)
  wc/1 -> Gain/1, Square/1, Gain1/1
  Gain/1 -> Discrete LESO 2nd Order/3(wo)
  t_warm/1 -> GreaterThan/2
  Digital Clock/1 -> GreaterThan/1
  GreaterThan/1 -> Switch/2
  y/1 -> Discrete LESO 2nd Order/4(y)
  Memory/1 -> Discrete LESO 2nd Order/1(z_in)
  Memory1/1 -> Sum4/2, Discrete LESO 2nd Order/5(u), Sum/2
  Rate Limit/1 -> Sum/1
  Sum/1 -> Magnitude Limit/1
  Sum4/1 -> Rate Limit/1
  Switch/1 -> Sum4/1
  Magnitude Limit/1 -> u/1, Memory1/1

== system flightController/Flight Controller - XBOX/LADRC - dX ==
  y : Inport
  r : Inport  Port=2
  Demux : Demux  Outputs=2
  Digital Clock : DigitalClock  SampleTime=Ts
  Discrete LESO 1st Order : MATLAB Function  TreatAsAtomicUnit=on
  Divide : Product  Inputs=*/
  GreaterThan : RelationalOperator  Operator=>  OutDataTypeStr=boolean  RndMeth=Simplest  InputSameDT=off
  Magnitude Limit : Saturate  UpperLimit=pi/8  LowerLimit=-pi/8  OutDataTypeStr=single
  Memory : Memory  InitialCondition=[0 0]'
  Memory1 : Memory
  Product : Product
  Rate Limit : Saturate  UpperLimit=1  LowerLimit=-1
  Sum : Sum  Inputs=|++
  Sum1 : Sum  Inputs=+-|
  Sum3 : Sum  Inputs=+-|
  Sum4 : Sum  Inputs=|+-
  Switch : Switch  Criteria=u2 ~= 0  Threshold=0.1  SaturateOnIntegerOverflow=off  InputSameDT=off
  b : Constant  Value=-60  OutDataTypeStr=single
  bw_o : Gain  Gain=3
  t_warm : Constant  Value=0.01
  u_ini : Constant  Value=0  OutDataTypeStr=single
  wc : Constant  Value=3  OutDataTypeStr=single
  u : Outport
  wires:
  Demux/1 -> Sum3/2  "z1"
  Product/1 -> Sum1/1
  Sum1/1 -> Divide/1  "u_0"
  Demux/2 -> Sum1/2  "z2"
  Magnitude Limit/1 -> u/1, Memory1/1  "u"
  Divide/1 -> Switch/1  "u"
  u_ini/1 -> Switch/3
  r/1 -> Sum3/1
  Sum3/1 -> Product/2
  b/1 -> Divide/2, Discrete LESO 1st Order/2(b)
  wc/1 -> Product/1, bw_o/1
  bw_o/1 -> Discrete LESO 1st Order/3(wo)
  t_warm/1 -> GreaterThan/2
  Digital Clock/1 -> GreaterThan/1
  GreaterThan/1 -> Switch/2
  y/1 -> Discrete LESO 1st Order/4(y)
  Switch/1 -> Sum4/1  "u"
  Discrete LESO 1st Order/1(z_out) -> Memory/1, Demux/1
  Memory/1 -> Discrete LESO 1st Order/1(z_in)
  Rate Limit/1 -> Sum/1
  Memory1/1 -> Discrete LESO 1st Order/5(u), Sum4/2, Sum/2
  Sum4/1 -> Rate Limit/1
  Sum/1 -> Magnitude Limit/1

== system flightController/Flight Controller - XBOX/LADRC - dY ==
  y : Inport
  r : Inport  Port=2
  Demux : Demux  Outputs=2
  Digital Clock : DigitalClock  SampleTime=Ts
  Discrete LESO 1st Order : MATLAB Function  TreatAsAtomicUnit=on
  Divide : Product  Inputs=*/
  GreaterThan : RelationalOperator  Operator=>  OutDataTypeStr=boolean  RndMeth=Simplest  InputSameDT=off
  Magnitude Limit : Saturate  UpperLimit=pi/8  LowerLimit=-pi/8  OutDataTypeStr=single
  Memory : Memory  InitialCondition=[0 0]'
  Memory1 : Memory
  Product : Product
  Rate Limit : Saturate  UpperLimit=1  LowerLimit=-1
  Sum : Sum  Inputs=|++
  Sum1 : Sum  Inputs=+-|
  Sum3 : Sum  Inputs=+-|
  Sum4 : Sum  Inputs=|+-
  Switch : Switch  Criteria=u2 ~= 0  Threshold=0.1  SaturateOnIntegerOverflow=off  InputSameDT=off
  b : Constant  Value=60  OutDataTypeStr=single
  bw_o : Gain  Gain=3
  t_warm : Constant  Value=0.01
  u_ini : Constant  Value=0  OutDataTypeStr=single
  wc : Constant  Value=3  OutDataTypeStr=single
  u : Outport
  wires:
  Demux/1 -> Sum3/2  "z1"
  Product/1 -> Sum1/1
  Sum1/1 -> Divide/1  "u_0"
  Demux/2 -> Sum1/2  "z2"
  Magnitude Limit/1 -> u/1, Memory1/1  "u"
  Divide/1 -> Switch/1  "u"
  u_ini/1 -> Switch/3
  r/1 -> Sum3/1
  Sum3/1 -> Product/2
  b/1 -> Divide/2, Discrete LESO 1st Order/2(b)
  wc/1 -> Product/1, bw_o/1
  bw_o/1 -> Discrete LESO 1st Order/3(wo)
  t_warm/1 -> GreaterThan/2
  Digital Clock/1 -> GreaterThan/1
  GreaterThan/1 -> Switch/2
  y/1 -> Discrete LESO 1st Order/4(y)
  Switch/1 -> Sum4/1  "u"
  Discrete LESO 1st Order/1(z_out) -> Memory/1, Demux/1
  Memory/1 -> Discrete LESO 1st Order/1(z_in)
  Rate Limit/1 -> Sum/1
  Memory1/1 -> Discrete LESO 1st Order/5(u), Sum4/2, Sum/2
  Sum4/1 -> Rate Limit/1
  Sum/1 -> Magnitude Limit/1

== system flightController/Flight Controller - XBOX/LADRC - dZ ==
  y : Inport
  r : Inport  Port=2
  Demux : Demux  Outputs=3
  Digital Clock : DigitalClock  SampleTime=Ts
  Discrete LESO 2nd Order : MATLAB Function  TreatAsAtomicUnit=on
  Divide : Product  Inputs=*/  OutDataTypeStr=single
  Gain : Gain  Gain=3  OutDataTypeStr=single
  Gain1 : Gain  Gain=2  OutDataTypeStr=single
  GreaterThan : RelationalOperator  Operator=>  OutDataTypeStr=boolean  RndMeth=Simplest  InputSameDT=off
  Magnitude Limit : Saturate  UpperLimit=4*Controller.totalThrustMaxRelative*Controller.motorsThrustPerMotorMax  LowerLimit=-4*Controller.totalThrustMaxRelative*Controller.motorsThrustPerMotorMax  OutDataTypeStr=single
  Memory : Memory  InitialCondition=[0 0 380]'
  Memory1 : Memory  InitialCondition=-0.6
  Product : Product  OutDataTypeStr=single
  Product1 : Product  OutDataTypeStr=single
  Rate Limit : Saturate  UpperLimit=0.025  LowerLimit=-0.025
  Square : Math  Operator=square
  Sum : Sum  Inputs=|++
  Sum1 : Sum  Inputs=+-|
  Sum2 : Sum  Inputs=|+-
  Sum3 : Sum  Inputs=+-|
  Sum4 : Sum  Inputs=|+-
  Switch : Switch  Criteria=u2 ~= 0  Threshold=0.1  SaturateOnIntegerOverflow=off  InputSameDT=off
  b : Constant  Value=800  OutDataTypeStr=single
  t_warm : Constant  Value=0  OutDataTypeStr=single
  u_ini : Constant  Value=0  OutDataTypeStr=single
  wc : Constant  Value=20  OutDataTypeStr=single
  u : Outport
  wires:
  Discrete LESO 2nd Order/1(z_out) -> Memory/1, Demux/1
  Demux/1 -> Sum3/2  "z1"
  Product/1 -> Sum1/1
  Sum1/1 -> Sum2/1  "u_0"
  Demux/3 -> Sum2/2  "z3"
  Sum2/1 -> Divide/1
  Square/1 -> Product/1
  Gain1/1 -> Product1/1
  Demux/2 -> Product1/2  "z2"
  Product1/1 -> Sum1/2
  Divide/1 -> Switch/1  "u"
  u_ini/1 -> Switch/3
  r/1 -> Sum3/1
  Sum3/1 -> Product/2
  b/1 -> Divide/2, Discrete LESO 2nd Order/2(b)
  wc/1 -> Gain/1, Square/1, Gain1/1
  Gain/1 -> Discrete LESO 2nd Order/3(wo)
  t_warm/1 -> GreaterThan/2
  Digital Clock/1 -> GreaterThan/1
  GreaterThan/1 -> Switch/2
  y/1 -> Discrete LESO 2nd Order/4(y)
  Memory/1 -> Discrete LESO 2nd Order/1(z_in)
  Memory1/1 -> Sum4/2, Discrete LESO 2nd Order/5(u), Sum/2
  Rate Limit/1 -> Sum/1
  Sum/1 -> Magnitude Limit/1
  Sum4/1 -> Rate Limit/1
  Switch/1 -> Sum4/1
  Magnitude Limit/1 -> u/1, Memory1/1

== system flightController/Flight Controller - XBOX/XBOX Input ==
  Bus Creator : BusCreator  Inputs=8
  Bus Creator1 : BusCreator  Inputs=11
  Constant : Constant  Value=[0 0 0 0 0 0 0 0]
  Dead Zone{,1..3} (4 alike) : DeadZone  LowerValue=-0.18  UpperValue=0.18
  Demux : Demux  Outputs=8
  Demux1 : Demux  Outputs=11
  Gain : Gain  Gain=-1
  Gain1 : Gain
  Joystick Input : vrlib/Joystick Input  joyid=1  adjustports=on  forcefeed=off
  Analog : Outport
  Buttons : Outport  Port=2
  wires:
  Demux1/4 -> Bus Creator1/4  "Y"
  Dead Zone/1 -> Bus Creator/1  "LStick-X"
  Demux1/9 -> Bus Creator1/9  "XBOX"
  Demux1/1 -> Bus Creator1/1  "A"
  Demux1/10 -> Bus Creator1/10  "LStick"
  Demux1/5 -> Bus Creator1/5  "LB"
  Demux/7 -> Bus Creator/7  "DPad-X"
  Joystick Input/2 -> Demux1/1
  Demux/5 -> Dead Zone3/1  "RStick-Y"
  Demux/4 -> Dead Zone2/1  "RStick-X"
  Dead Zone2/1 -> Bus Creator/4  "RStick-X"
  Demux/3 -> Bus Creator/3  "LT"
  Demux/8 -> Bus Creator/8  "DPad-Y"
  Joystick Input/1 -> Demux/1
  Demux/6 -> Bus Creator/6  "RT"
  Dead Zone1/1 -> Gain1/1  "LStick-Y"
  Demux/1 -> Dead Zone/1  "LStick-X"
  Bus Creator1/1 -> Buttons/1  "Buttons"
  Gain/1 -> Bus Creator/5  "RStick-Y"
  Demux/2 -> Dead Zone1/1  "LStick-Y"
  Bus Creator/1 -> Analog/1  "Analog"
  Demux1/3 -> Bus Creator1/3  "X"
  Demux1/6 -> Bus Creator1/6  "RB"
  Demux1/7 -> Bus Creator1/7  "Back"
  Demux1/11 -> Bus Creator1/11  "RStick"
  Demux1/2 -> Bus Creator1/2  "B"
  Demux1/8 -> Bus Creator1/8  "Start"
  Dead Zone3/1 -> Gain/1  "RStick-Y"
  Gain1/1 -> Bus Creator/2  "LStick-Y"

== system flightController/Flight Controller - XBOX/thrustsToMotorCommands ==
  thrusts_refin : Inport
  1 : Constant  OutDataTypeStr=single
  2 : Constant  Value=-1  OutDataTypeStr=single
  3 : Constant  OutDataTypeStr=single
  Digital Clock : DigitalClock  SampleTime=Ts
  GreaterThan : RelationalOperator  Operator=>  OutDataTypeStr=boolean  RndMeth=Simplest  InputSameDT=off
  MotorDirections : Gain  Gain=[1 -1 1 -1]
  Mux : Mux
  Product : Product  OutDataTypeStr=single
  Saturation5 : Saturate  UpperLimit=Vehicle.Motor.maxLimit  LowerLimit=Vehicle.Motor.minLimit
  Switch : Switch  Criteria=u2 ~= 0  Threshold=0.1  SaturateOnIntegerOverflow=off  InputSameDT=off
  ThrustToMotorCommand : Gain  Gain=-Vehicle.Motor.thrustToMotorCommand
  t_warm : Constant  Value=10  OutDataTypeStr=single
  motors_cmdout : Outport  VectorParamsAs1DForOutWhenUnconnected=off
  wires:
  Saturation5/1 -> Product/2, MotorDirections/1
  MotorDirections/1 -> Switch/3
  ThrustToMotorCommand/1 -> Saturation5/1
  thrusts_refin/1 -> ThrustToMotorCommand/1
  Product/1 -> Switch/1
  Switch/1 -> motors_cmdout/1
  GreaterThan/1 -> Switch/2
  Digital Clock/1 -> GreaterThan/1
  t_warm/1 -> GreaterThan/2
  1/1 -> Mux/3
  2/1 -> Mux/2, Mux/4
  3/1 -> Mux/1
  Mux/1 -> Product/1

== system flightController/Flight Controller1/ControlMixer ==
  tau_pitch : Inport
  tau_roll : Inport  Port=2
  tau_yaw : Inport  Port=3
  totalThrust : Inport  Port=4
  Mux2 : Mux
  Product : Product  Multiplication=Matrix(*)  RndMeth=Zero
  TorqueTotalThrustToThrustPerMotor : Constant  Value=Controller.Q2Ts  OutDataTypeStr=single
  thrusts_refout : Outport  VectorParamsAs1DForOutWhenUnconnected=off
  wires:
  Product/1 -> thrusts_refout/1
  tau_roll/1 -> Mux2/4
  tau_pitch/1 -> Mux2/3
  tau_yaw/1 -> Mux2/2
  totalThrust/1 -> Mux2/1
  TorqueTotalThrustToThrustPerMotor/1 -> Product/1
  Mux2/1 -> Product/2

== system flightController/Flight Controller1/LADRC - Pitch ==
  y : Inport
  r : Inport  Port=2
  Demux : Demux  Outputs=3
  Digital Clock : DigitalClock  SampleTime=Ts
  Discrete-Time Integrator : DiscreteIntegrator  InitialCondition=[0 0 0]'  SampleTime=Ts  OutDataTypeStr=single  ICPrevOutput=DiscIntNeverNeededParam  ICPrevScaledInput=DiscIntNeverNeededParam
  Divide : Product  Inputs=*/  OutDataTypeStr=single
  Gain1 : Gain  Gain=2  OutDataTypeStr=single
  GreaterThan : RelationalOperator  Operator=>  OutDataTypeStr=boolean  RndMeth=Simplest  InputSameDT=off
  LESO : MATLAB Function  TreatAsAtomicUnit=on
  Product : Product  OutDataTypeStr=single
  Product1 : Product  OutDataTypeStr=single
  SaturationThrust : Saturate  UpperLimit=4*Controller.totalThrustMaxRelative*Controller.motorsThrustPerMotorMax  LowerLimit=-4*Controller.totalThrustMaxRelative*Controller.motorsThrustPerMotorMax  OutDataTypeStr=single
  Square : Math  Operator=square
  Sum1 : Sum  Inputs=+-|
  Sum2 : Sum  Inputs=|+-
  Sum3 : Sum  Inputs=+-|
  Switch : Switch  Criteria=u2 ~= 0  Threshold=0.1  SaturateOnIntegerOverflow=off  InputSameDT=off
  b : Constant  Value=10000  OutDataTypeStr=single
  t_warm : Constant  Value=0.1  OutDataTypeStr=single
  u_ini : Constant  Value=0  OutDataTypeStr=single
  wc : Constant  Value=12  OutDataTypeStr=single
  wo : Constant  Value=40  OutDataTypeStr=single
  u : Outport
  wires:
  LESO/1(z_dot) -> Discrete-Time Integrator/1
  Discrete-Time Integrator/1 -> LESO/1(z), Demux/1
  Demux/1 -> Sum3/2  "z1"
  Product/1 -> Sum1/1
  Sum1/1 -> Sum2/1  "u_0"
  Demux/3 -> Sum2/2  "z3"
  Sum2/1 -> Divide/1
  Square/1 -> Product/1
  Gain1/1 -> Product1/1
  Demux/2 -> Product1/2  "z2"
  Product1/1 -> Sum1/2
  SaturationThrust/1 -> LESO/5(u), u/1  "u"
  Switch/1 -> SaturationThrust/1
  Divide/1 -> Switch/1  "u"
  u_ini/1 -> Switch/3
  r/1 -> Sum3/1
  Sum3/1 -> Product/2
  b/1 -> LESO/3(b), Divide/2
  wc/1 -> Gain1/1, Square/1
  wo/1 -> LESO/2(wo)
  t_warm/1 -> GreaterThan/2
  Digital Clock/1 -> GreaterThan/1
  GreaterThan/1 -> Switch/2
  y/1 -> LESO/4(y)
